simulink model "MM_dpt"  (R2021b)
settings: Solver=VariableStepAuto  StartTime=0.0  StopTime=1  RelTol=1e-3
undefined symbols (not defined in the file): Jn, ke, km, ku, R, Te
settings Model: Creator=vkad  LastModifiedBy=vkad

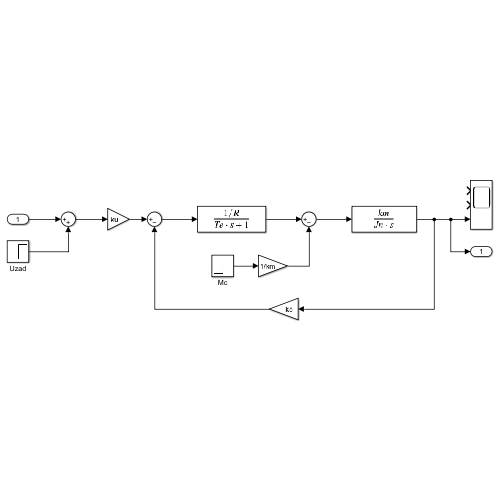
[thumbnail: Simulink's stored preview of the top-level diagram]
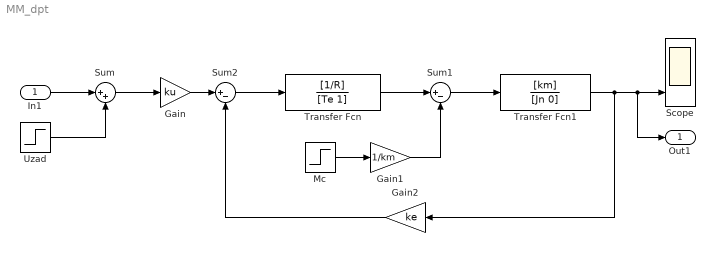
== system MM_dpt ==
  In1 : Inport
  Gain : Gain  Gain=ku
  Gain1 : Gain  Gain=1/km
  Gain2 : Gain  Gain=ke
  Mc : Step  Time=0  SampleTime=0
  Scope : Scope  NumInputPorts=3
  Sum : Sum  Inputs=|++
  Sum1 : Sum  Inputs=|+-
  Sum2 : Sum  Inputs=|+-
  Transfer Fcn : TransferFcn  Numerator=[1/R]  Denominator=[Te 1]
  Transfer Fcn1 : TransferFcn  Numerator=[km]  Denominator=[Jn 0]
  Uzad : Step  Time=0  After=3  SampleTime=0
  Out1 : Outport
  wires:
  Sum/1 -> Gain/1
  Transfer Fcn/1 -> Sum1/1
  Sum1/1 -> Transfer Fcn1/1
  Gain1/1 -> Sum1/2
  Mc/1 -> Gain1/1
  In1/1 -> Sum/1
  Uzad/1 -> Sum/2
  Transfer Fcn1/1 -> Out1/1, Scope/3, Gain2/1
  Gain/1 -> Sum2/1
  Sum2/1 -> Transfer Fcn/1
  Gain2/1 -> Sum2/2
